simulink model "simplePid"  (R2020a)
settings: Solver=VariableStepAuto  StartTime=0.0  StopTime=10.0  RelTol=1e-3
libraries: robotlib x9
settings Model: Creator=user  LastModifiedBy=user

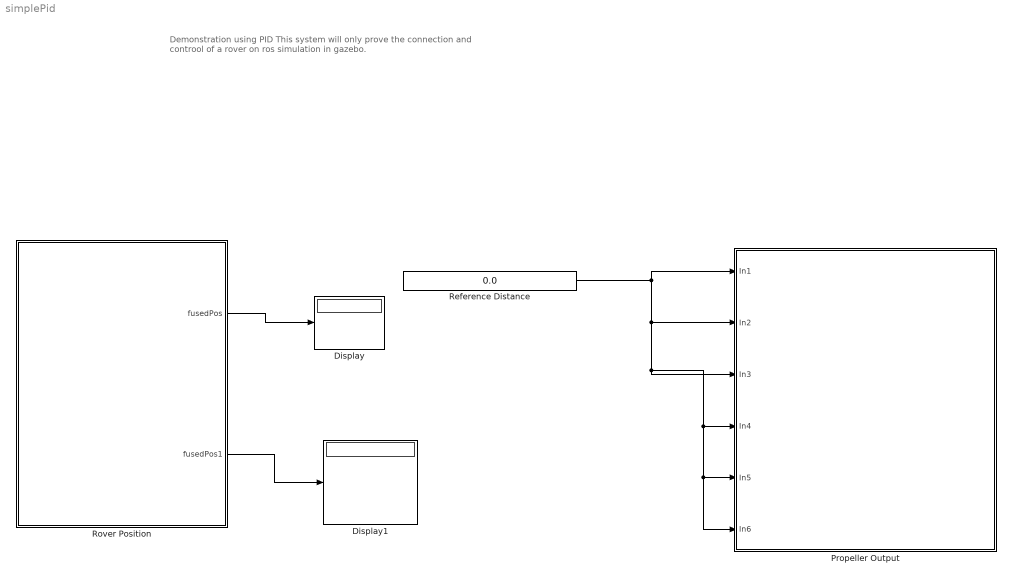
== system simplePid ==
  note: Demonstration using PID
      |
      | This system will only prove the connection and controol of a rover on ros simulation in gazebo.
  Display : Display
  Display1 : Display
  Propeller Output : Subsystem
  Reference Distance : Constant  Value=0.0
  Rover Position : Subsystem
  wires:
  Reference Distance/1 -> Propeller Output/1(In1), Propeller Output/6(In6), Propeller Output/5(In5), Propeller Output/4(In4), Propeller Output/3(In3), Propeller Output/2(In2)
  Rover Position/1(fusedPos) -> Display/1
  Rover Position/2(fusedPos1) -> Display1/1

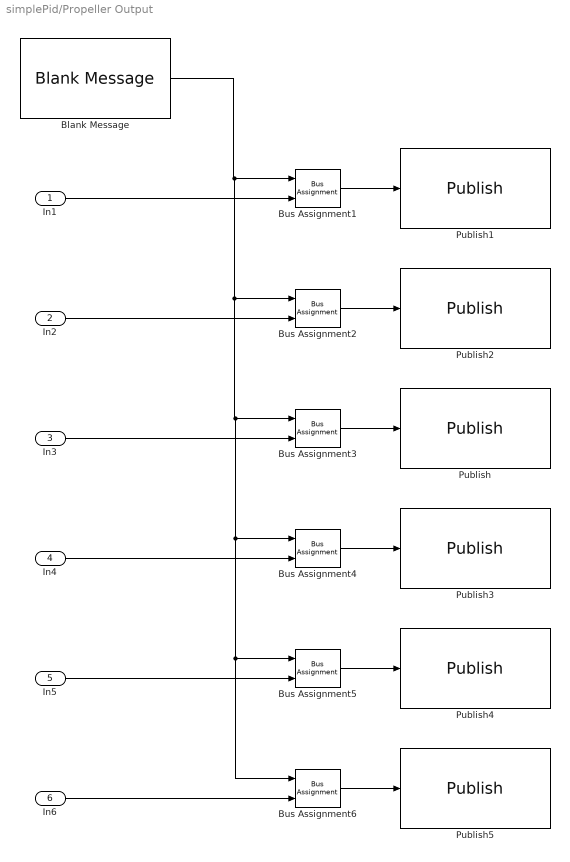
== system simplePid/Propeller Output ==
  In1 : Inport
  In2 : Inport  Port=2
  In3 : Inport  Port=3
  In4 : Inport  Port=4
  In5 : Inport  Port=5
  In6 : Inport  Port=6
  Blank Message : robotlib/Blank Message  messageClass=Message  entityType=uuv_gazebo_ros_plugins_msgs/FloatStamped  messageType=uuv_gazebo_ros_plugins_msgs/FloatStamped  SampleTime=inf
  Bus Assignment{1..6} (6 alike) : BusAssignment  AssignedSignals=Data
  Publish : robotlib/Publish  topicSource=Select from ROS network  topic=/bluerov2/thrusters/2/input  messageType=uuv_gazebo_ros_plugins_msgs/FloatStamped  messageQueueLength=1
  Publish1 : robotlib/Publish  topicSource=Select from ROS network  topic=/bluerov2/thrusters/0/input  messageType=uuv_gazebo_ros_plugins_msgs/FloatStamped  messageQueueLength=1
  Publish2 : robotlib/Publish  topicSource=Select from ROS network  topic=/bluerov2/thrusters/1/input  messageType=uuv_gazebo_ros_plugins_msgs/FloatStamped  messageQueueLength=1
  Publish3 : robotlib/Publish  topicSource=Select from ROS network  topic=/bluerov2/thrusters/3/input  messageType=uuv_gazebo_ros_plugins_msgs/FloatStamped  messageQueueLength=1
  Publish4 : robotlib/Publish  topicSource=Select from ROS network  topic=/bluerov2/thrusters/4/input  messageType=uuv_gazebo_ros_plugins_msgs/FloatStamped  messageQueueLength=1
  Publish5 : robotlib/Publish  topicSource=Select from ROS network  topic=/bluerov2/thrusters/5/input  messageType=uuv_gazebo_ros_plugins_msgs/FloatStamped  messageQueueLength=1
  wires:
  Bus Assignment5/1 -> Publish4/1
  Bus Assignment4/1 -> Publish3/1
  Bus Assignment3/1 -> Publish/1
  Bus Assignment2/1 -> Publish2/1
  Bus Assignment1/1 -> Publish1/1
  Bus Assignment6/1 -> Publish5/1
  Blank Message/1 -> Bus Assignment6/1, Bus Assignment5/1, Bus Assignment4/1, Bus Assignment3/1, Bus Assignment2/1, Bus Assignment1/1
  In1/1 -> Bus Assignment1/2
  In2/1 -> Bus Assignment2/2
  In3/1 -> Bus Assignment3/2
  In4/1 -> Bus Assignment4/2
  In5/1 -> Bus Assignment5/2
  In6/1 -> Bus Assignment6/2

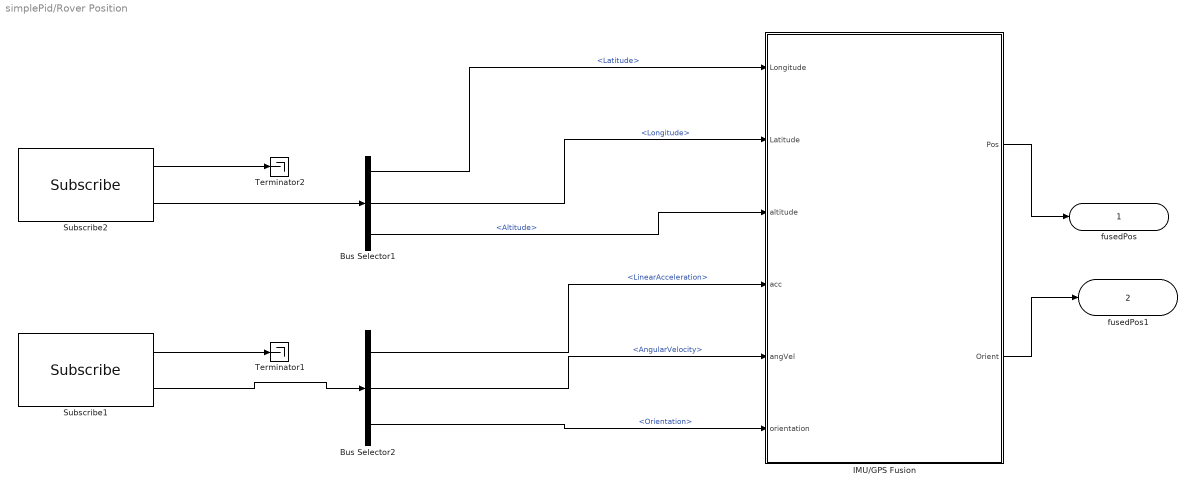
== system simplePid/Rover Position ==
  Bus Selector1 : BusSelector  OutputSignals=Latitude,Longitude,Altitude
  Bus Selector2 : BusSelector  OutputSignals=LinearAcceleration,AngularVelocity,Orientation
  IMU/GPS Fusion : MATLAB Function  TreatAsAtomicUnit=on
  Subscribe1 : robotlib/Subscribe  topicSource=Select from ROS network  topic=/bluerov2/imu  messageType=sensor_msgs/Imu  sampleTime=-1  messageQueueLength=1
  Subscribe2 : robotlib/Subscribe  topicSource=Select from ROS network  topic=/bluerov2/gps  messageType=sensor_msgs/NavSatFix  sampleTime=-1  messageQueueLength=1
  Terminator1 : Terminator
  Terminator2 : Terminator
  fusedPos : Outport
  fusedPos1 : Outport  Port=2
  wires:
  Subscribe1/2 -> Bus Selector2/1
  Subscribe1/1 -> Terminator1/1
  Subscribe2/1 -> Terminator2/1
  Subscribe2/2 -> Bus Selector1/1
  Bus Selector1/1 -> IMU/GPS Fusion/1(Longitude)  "<Latitude>"
  Bus Selector1/2 -> IMU/GPS Fusion/2(Latitude)  "<Longitude>"
  Bus Selector1/3 -> IMU/GPS Fusion/3(altitude)  "<Altitude>"
  IMU/GPS Fusion/1(Pos) -> fusedPos/1
  IMU/GPS Fusion/2(Orient) -> fusedPos1/1
  Bus Selector2/1 -> IMU/GPS Fusion/4(acc)  "<LinearAcceleration>"
  Bus Selector2/2 -> IMU/GPS Fusion/5(angVel)  "<AngularVelocity>"
  Bus Selector2/3 -> IMU/GPS Fusion/6(orientation)  "<Orientation>"

== matlab function simplePid/Rover Position/IMU//GPS Fusion ==
  data: Pos output; Orient output; Longitude input; Latitude input; altitude input; acc input; angVel input; orientation input
function [Pos, Orient]= fcn(Longitude, Latitude,altitude,acc,angVel,orientation)
imuFs = 100;
Rmag = 0.09; % Magnetometer measurement noise
Rvel = 0.01; % GPS Velocity measurement noise
Rpos = 2.56; % GPS Position measurement noise

refloc = [-56.7189766963 -3.515625 -0.0996294077486];
fusionfilter = insfilterMARG;
fusionfilter.IMUSampleRate = imuFs;
fusionfilter.ReferenceLocation = refloc;

imu = imuSensor('accel-gyro-mag', 'SampleRate', imuFs);
[accel, gyro, mag] = imu([acc.X,acc.Y,acc.Z],[angVel.X,angVel.Y,angVel.Z],quaternion(orientation.X,orientation.Y,orientation.Z,orientation.W));

predict(fusionfilter, accel, gyro);
fusegps(fusionfilter, [Latitude Longitude altitude], Rpos);
fusemag(fusionfilter, mag, Rmag);



[Pos, OrientQuad] = pose(fusionfilter);
Orient = compact(OrientQuad);
